simulink model "EX004_FCHEVgasExchange"  (R2023a)
settings: Solver=ode23tb  StartTime=0.0  StopTime=20e3  MaxStep=1e-1  RelTol=1e-4
libraries: component_lib x23, slpidlib x4, simulink x1, base_lib x1
settings Model: Creator=maxjo65  LastModifiedBy=maxjo
settings OptimizationCC: ReuseModelBlockBuffer=off
settings DebuggingCC: UnconnectedInputMsg=warning  UnconnectedOutputMsg=warning  UnconnectedLineMsg=warning
settings ModelReferenceCC: EnableRefExpFcnMdlSchedulingChecks=on
settings RTWCC: DLArmComputeVersion=19.05

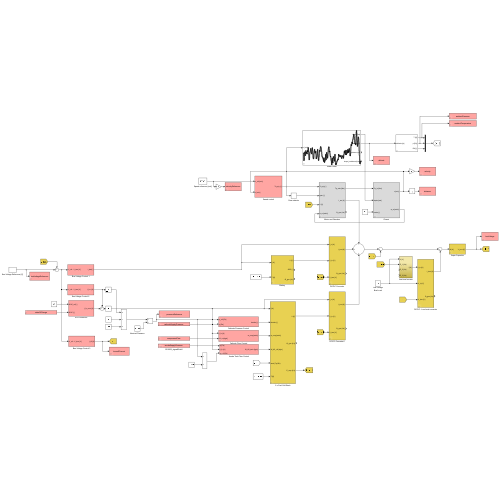
[thumbnail: Simulink's stored preview of the top-level diagram]
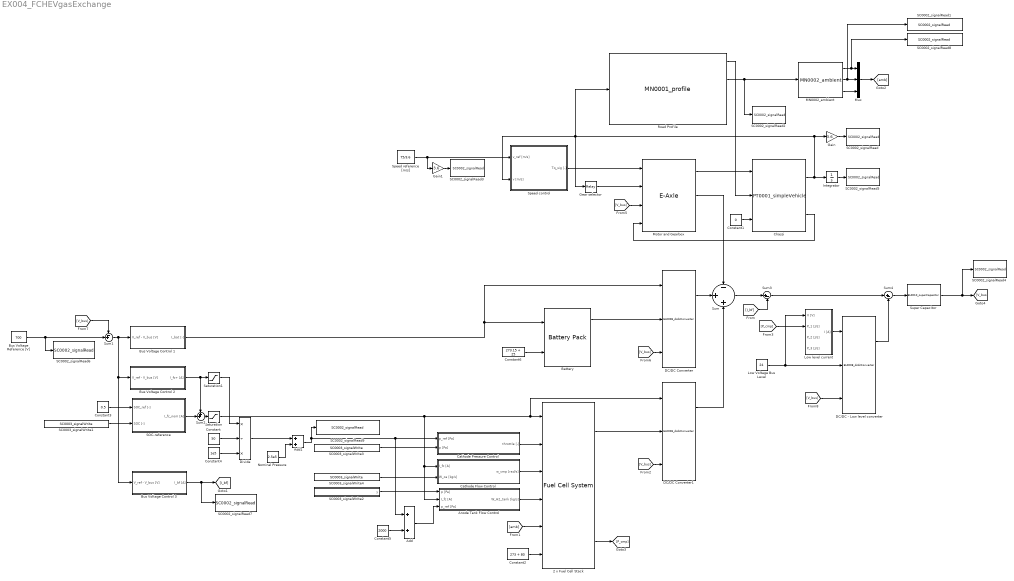
== system EX004_FCHEVgasExchange ==
  2 x Fuel Cell Stack : component_lib/Fuel Cell System  n_st=2  n=375
  Add : Sum
  Add1 : Sum
  Anode Tank Flow Control : Subsystem  mask{n_cell=375}
      mask prompts: n_cell "Cells [-]"
  Battery : component_lib/Battery Pack  SOC_0=0.5  Nx=120  Ny=180
  Bus Voltage Control 1 : Subsystem
  "Bus Voltage Control 2 " : Subsystem
  Bus Voltage Control 3 : Subsystem
  Bus Voltage Reference [V] : Constant  Value=700
  Cathode Flow Control : Subsystem  mask{lambda_O2_ref=2, n_cell=375}
      mask prompts: lambda_O2_ref "Oxygen stoich. reference [-]:"; n_cell "Cells [-]:"
  Cathode Pressure Control : Subsystem
  Chassi : component_lib/Powertrain/PT0001_simpleVehicle  m=40e3  r_w=0.5  A_f=10  C_d=0.5  rho_air=1.225  c_r0=0.0060  c_r1=2.3e-7  gain=600  v0=75/3.6  x0=0
  Constant : Constant  Value=50
  Constant1 : Constant  Value=0
  Constant2 : Constant  Value=273 + 80
  Constant3 : Constant  Value=0.5
  Constant4 : Constant  Value=1e5
  Constant5 : Constant  Value=2000
  Constant6 : Constant  Value=273.15 + 25
  DC/DC - Low level converter : component_lib/Electrochemistry/EL0008_dcdcConverter  eta_up=0.99  eta_down=0.99
  DC/DC Converter : component_lib/Electrochemistry/EL0008_dcdcConverter  eta_up=0.99  eta_down=0.99
  DC/DC Converter1 : component_lib/Electrochemistry/EL0008_dcdcConverter  eta_up=0.99  eta_down=0.99
  Divide : Product  Inputs=*/*
  Gain : Gain  Gain=3.6
  Gain1 : Gain  Gain=3.6
  Gear selector : Relay  OnSwitchValue=22  OffSwitchValue=21.5  OnOutputValue=4  OffOutputValue=3
  Integrator : Integrator
  Low Voltage Bus Level : Constant  Value=24
  Low level current : Subsystem
  MN0002_ambient : component_lib/Mission/MN0002_ambient  p_0=1.01e5  T_0=273 + 20  RH_0=0.05
  Motor and Gearbox : component_lib/E-Axle  n=3  V_nom=700
  Mux : Mux  Inputs=3
  Nominal Pressure : Constant  Value=2.5e5
  Road Profile : component_lib/Mission/MN0001_profile  profile=Sodertalje_Norrkoping.mat  x0=0  N_lookahead=100
  SC0002_signalRead : component_lib/Data & Control/SC0002_signalRead  SigName=velocity
  SC0002_signalRead1 : component_lib/Data & Control/SC0002_signalRead  SigName=ambientPressure
  SC0002_signalRead2 : component_lib/Data & Control/SC0002_signalRead  SigName=altitude
  SC0002_signalRead3 : component_lib/Data & Control/SC0002_signalRead  SigName=velocityReference
  SC0002_signalRead4 : component_lib/Data & Control/SC0002_signalRead  SigName=busVoltage
  SC0002_signalRead5 : component_lib/Data & Control/SC0002_signalRead  SigName=distance
  SC0002_signalRead6 : component_lib/Data & Control/SC0002_signalRead  SigName=busVoltageReference
  SC0002_signalRead7 : component_lib/Data & Control/SC0002_signalRead  SigName=burnoffCurrent
  SC0002_signalRead8 : component_lib/Data & Control/SC0002_signalRead  SigName=ambientTemperature
  SC0002_signalRead9 : component_lib/Data & Control/SC0002_signalRead  SigName=pressureReference
  SC0003_signalWrite1 : component_lib/Data & Control/SC0003_signalWrite  SigName=stateOfCharge
  SC0003_signalWrite2 : Subsystem  AncestorBlock=component_lib/Data & Control/SC0003_signalWrite  mask{SigName=anodeSupplyPressure}
      mask prompts: SigName "Signal identifier:"
      mask init:
      | % set signal name in goto tag
      | set_param([gcb, '/', 'From'], 'GotoTag', SigName)
      settings: LibrarySourceBlock=component_lib/Data & Control/SC0003_signalWrite
      mask Display: disp(SigName)
  SC0003_signalWrite3 : component_lib/Data & Control/SC0003_signalWrite  SigName=cathodeSupplyPressure
  SC0003_signalWrite4 : component_lib/Data & Control/SC0003_signalWrite  SigName=compressorFlow
  SOC-reference : Subsystem
  Saturation : Saturate  UpperLimit=600  LowerLimit=20
  Saturation1 : Saturate  UpperLimit=50  LowerLimit=0
  Speed control : Subsystem
  Speed reference [m/s] : Constant  Value=75/3.6
  Sum : Sum  Inputs=-++
  Sum1 : Sum  Inputs=-+|
  Sum2 : Sum  Inputs=++|
  Sum3 : Sum  Inputs=|+-
  Sum4 : Sum  Inputs=|+-
  Super Capacitor : component_lib/Electrochemistry/EL0010_superCapacitor  C=1  V_bus0=700
  wires:
  Motor and Gearbox/1 -> Chassi/1
  Chassi/2 -> Motor and Gearbox/4
  Road Profile/1 -> Chassi/2
  Chassi/1 -> Integrator/1, Gain/1, Speed control/2(v [m/s]), Road Profile/1, Gear selector/1
  Speed reference [m/s]/1 -> Gain1/1, Speed control/1(v_ref [m/s])
  Speed control/1(Tq_sig [-]) -> Motor and Gearbox/1
  Gear selector/1 -> Motor and Gearbox/2
  Integrator/1 -> SC0002_signalRead5/1
  Gain/1 -> SC0002_signalRead/1
  Road Profile/2 -> MN0002_ambient/1, SC0002_signalRead2/1
  Gain1/1 -> SC0002_signalRead3/1
  Super Capacitor/1 -> SC0002_signalRead4/1, [V_bus]
  Constant1/1 -> Chassi/3
  Battery/1 -> DC/DC Converter/2
  DC/DC Converter/1 -> Sum/2
  Motor and Gearbox/2 -> Sum/1
  Bus Voltage Control 1/1(I_bat [-]) -> DC/DC Converter/1, Battery/1
  DC/DC Converter1/1 -> Sum/3
  Bus Voltage Reference [V]/1 -> Sum1/2, SC0002_signalRead6/1
  Constant3/1 -> SOC-reference/1(SOC_ref [-])
  Sum1/1 -> Bus Voltage Control 3/1(V_ref - V_bus [V]), "Bus Voltage Control 2 "/1(V_ref - V_bus [V]), Bus Voltage Control 1/1(V_ref - V_bus [V])
  Sum2/1 -> Saturation/1
  "Bus Voltage Control 2 "/1(I_fc+ [A]) -> Saturation1/1, Sum2/1
  SOC-reference/1(I_fc_nom [A]) -> Sum2/2
  Sum/1 -> Sum3/1
  Bus Voltage Control 3/1(I_bf [A]) -> SC0002_signalRead7/1, [I_bf]
  [I_bf] -> Sum3/2
  MN0002_ambient/3 -> Mux/3
  Mux/1 -> [amb]
  2 x Fuel Cell Stack/1 -> DC/DC Converter1/2
  2 x Fuel Cell Stack/3 -> [P_cmp]
  Sum3/1 -> Sum4/1
  Sum4/1 -> Super Capacitor/1
  DC/DC - Low level converter/1 -> Sum4/2
  [P_cmp] -> Low level current/2(P_1 [J/s])
  Low Voltage Bus Level/1 -> Low level current/1(V [V]), DC/DC - Low level converter/2
  [V_bus] -> Motor and Gearbox/3
  [V_bus] -> Sum1/1
  Cathode Flow Control/1(w_cmp [rad/s]) -> 2 x Fuel Cell Stack/3
  SC0003_signalWrite4/1 -> Cathode Flow Control/2(W_ca [kg/s])
  Cathode Pressure Control/1(throttle [-]) -> 2 x Fuel Cell Stack/2
  SC0003_signalWrite3/1 -> Cathode Pressure Control/2(p [Pa])
  SC0003_signalWrite2/1(y) -> Anode Tank Flow Control/1(p [Pa])
  Add1/1 -> Add/1, Cathode Pressure Control/1(p_ref [Pa]), SC0002_signalRead9/1
  Anode Tank Flow Control/1(W_H2_tank [kg/s]) -> 2 x Fuel Cell Stack/4
  Add/1 -> Anode Tank Flow Control/3(p_ref [Pa])
  Constant5/1 -> Add/2
  Saturation/1 -> Anode Tank Flow Control/2(I_fc [A]), Cathode Flow Control/1(I_fc [A]), DC/DC Converter1/1, 2 x Fuel Cell Stack/1
  Constant2/1 -> 2 x Fuel Cell Stack/6
  [amb] -> 2 x Fuel Cell Stack/5
  SC0003_signalWrite1/1 -> SOC-reference/2(SOC [-])
  MN0002_ambient/2 -> Mux/2, SC0002_signalRead1/1
  MN0002_ambient/1 -> SC0002_signalRead8/1, Mux/1
  Constant/1 -> Divide/2
  Constant4/1 -> Divide/3
  Nominal Pressure/1 -> Add1/2
  Saturation1/1 -> Divide/1
  Divide/1 -> Add1/1
  [V_bus] -> DC/DC Converter/3
  Constant6/1 -> Battery/2
  [V_bus] -> DC/DC Converter1/3
  Low level current/1(I [A]) -> DC/DC - Low level converter/1
  [V_bus] -> DC/DC - Low level converter/3

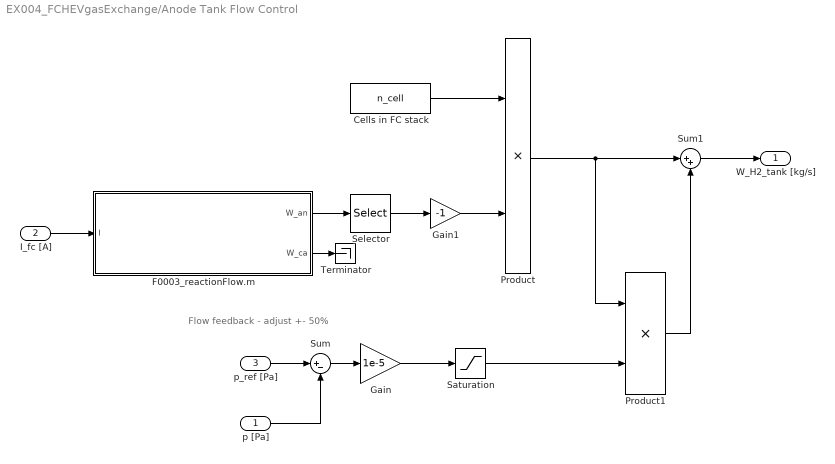
== system EX004_FCHEVgasExchange/Anode Tank Flow Control ==
  note: Flow feedback - adjust +- 50%
  p [Pa] : Inport
  I_fc [A] : Inport  Port=2
  p_ref [Pa] : Inport  Port=3
  Cells in FC stack : Constant  Value=n_cell
  F0003_reactionFlow.m : MATLAB Function  TreatAsAtomicUnit=on
  Gain : Gain  Gain=1e-5
  Gain1 : Gain  Gain=-1
  Product : Product
  Product1 : Product
  Saturation : Saturate
  Selector : Selector  InputPortWidth=4  IndexOptions=Index vector (dialog)  Indices=1  OutputSizes=1
  Sum : Sum  Inputs=|+-
  Sum1 : Sum  Inputs=|++
  Terminator : Terminator
  W_H2_tank [kg/s] : Outport
  wires:
  Product1/1 -> Sum1/2
  Sum/1 -> Gain/1
  Sum1/1 -> W_H2_tank [kg/s]/1
  Product/1 -> Product1/1, Sum1/1
  p [Pa]/1 -> Sum/2
  p_ref [Pa]/1 -> Sum/1
  Cells in FC stack/1 -> Product/1
  F0003_reactionFlow.m/2(W_ca) -> Terminator/1
  I_fc [A]/1 -> F0003_reactionFlow.m/1(I)
  F0003_reactionFlow.m/1(W_an) -> Selector/1
  Selector/1 -> Gain1/1
  Gain1/1 -> Product/2
  Gain/1 -> Saturation/1
  Saturation/1 -> Product1/2

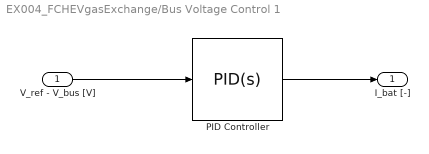
== system EX004_FCHEVgasExchange/Bus Voltage Control 1 ==
  V_ref - V_bus [V] : Inport
  PID Controller : slpidlib/PID Controller  Controller=PID  Form=Parallel  TimeDomain=Continuous-time  UseExternalTs=off  SampleTime=-1  IntegratorMethod=Forward Euler  FilterMethod=Forward Euler  ControllerParametersSource=internal  P=1e2  I=1  UseKiTs=off  D=0  N=100  UseFilter=on  TunerSelectOption=Transfer Function Based (PID Tuner App)  ZeroCross=off  InitialConditionSource=internal  InitialConditionForIntegrator=0  InitialConditionForFilter=0  DifferentiatorICPrevScaledInput=0  ExternalReset=none  TrackingMode=off  Kt=1  LimitOutput=on  SatLimitsSource=internal  UpperSaturationLimit=350  LowerSaturationLimit=-350  LinearizeAsGain=on  AntiWindupMode=clamping  Kb=1  LimitIntegrator=off  UpperIntegratorSaturationLimit=inf  LowerIntegratorSaturationLimit=-inf  POutMin=[]  POutMax=[]  IOutMin=[]  IOutMax=[]  DOutMin=[]  DOutMax=[]  NOutMin=[]  NOutMax=[]  SumOutMin=[]  SumOutMax=[]  SaturationOutMin=[]  SaturationOutMax=[]  PParamMin=[]  PParamMax=[]  IParamMin=[]  IParamMax=[]  DParamMin=[]  DParamMax=[]  NParamMin=[]  NParamMax=[]  KbParamMin=[]  KbParamMax=[]  KtParamMin=[]  KtParamMax=[]  KbOutMin=[]  KbOutMax=[]  KtOutMin=[]  KtOutMax=[]  IntegratorOutMin=[]  IntegratorOutMax=[]  FilterOutMin=[]  FilterOutMax=[]  SumI1OutMin=[]  SumI1OutMax=[]  SumI2OutMin=[]  SumI2OutMax=[]  SumI3OutMin=[]  SumI3OutMax=[]  SumI4OutMin=[]  SumI4OutMax=[]  SumDOutMin=[]  SumDOutMax=[]  DifferentiatorOutMin=[]  DifferentiatorOutMax=[]  FilterDiffOutCoefMin=[]  FilterDiffOutCoefMax=[]  ReciprocalOutMin=[]  ReciprocalOutMax=[]  SumDenOutMin=[]  SumDenOutMax=[]  SumNumOutMin=[]  SumNumOutMax=[]  DivideOutMin=[]  DivideOutMax=[]  UdiffTsProdOutMin=[]  UdiffTsProdOutMax=[]  NTsProdOutMin=[]  NTsProdOutMax=[]  UintegralTsProdOutMin=[]  UintegralTsProdOutMax=[]  UngainTsProdOutMin=[]  UngainTsProdOutMax=[]  ClampingZeroOutDataTypeStr=Inherit: Inherit via back propagation  ClampingZeroOutMin=[]  ClampingZeroOutMax=[]  FilterDenConstantOutDataTypeStr=Inherit: Inherit via back propagation  FilterDenConstantOutMin=[]  FilterDenConstantOutMax=[]  PCopyOutDataTypeStr=Inherit: Inherit via back propagation  PCopyOutMin=[]  PCopyOutMax=[]  NCopyOutDataTypeStr=Inherit: Inherit via back propagation  NCopyOutMin=[]  NCopyOutMax=[]  IntegratorContinuousStateAttributes=''  IntegratorStateMustResolveToSignalObject=off  IntegratorRTWStateStorageClass=Auto  FilterContinuousStateAttributes=''  FilterStateMustResolveToSignalObject=off  FilterRTWStateStorageClass=Auto  ParallelPVariant=InternalParameters  IdealPVariant=Disabled  IVariant=InternalParameters  DVariant=InternalParameters  IntegratorVariant=Continuous  SatVariant=Enabled  AWVariant=ContClampingParallel  PCopyVariant=Disabled  TRVariant=Disabled  FdbkBlocksVariant=Forward  IdealPFdbkVariant=Disabled  SatFdbkVariant=Disabled  DerivativeFilterVariant=ContFilter  NVariant=InternalParameters  NCopyVariant=Disabled  FilterICVariant=InternalICsFilter  IntegratorICVariant=InternalICs  ExternalResetVariant=Disabled  TRSumVariant=Passthrough  SumFdbkVariant=Disabled  SumVariant=Sum_PID  TsampFilterVariant=InternalTs  TsampNgainVariant=Passthrough  TsampIntegralVariant=Disabled_SignalSpec  ExternalSaturationOutDataTypeStr=Inherit: Same as second input
  I_bat [-] : Outport
  wires:
  PID Controller/1 -> I_bat [-]/1
  V_ref - V_bus [V]/1 -> PID Controller/1

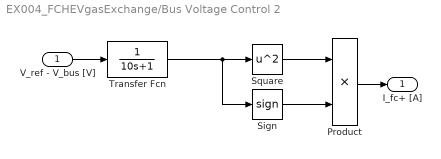
== system EX004_FCHEVgasExchange/Bus Voltage Control 2  ==
  V_ref - V_bus [V] : Inport
  Product : Product
  Sign : Signum
  Square : Math  Operator=square
  Transfer Fcn : TransferFcn  Denominator=[10 1]
  I_fc+ [A] : Outport
  wires:
  Sign/1 -> Product/2
  Transfer Fcn/1 -> Sign/1, Square/1
  Square/1 -> Product/1
  V_ref - V_bus [V]/1 -> Transfer Fcn/1
  Product/1 -> I_fc+ [A]/1

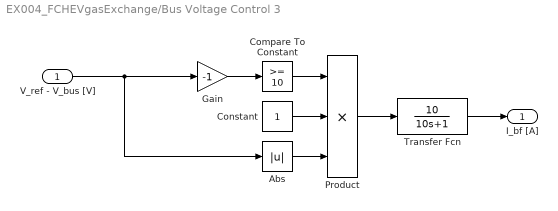
== system EX004_FCHEVgasExchange/Bus Voltage Control 3 ==
  V_ref - V_bus [V] : Inport
  Abs : Abs  SaturateOnIntegerOverflow=off
  Compare To Constant : simulink/Logic and Bit Operations/Compare To Constant  relop=>=  const=10  OutDataTypeStr=boolean
  Constant : Constant
  Gain : Gain  Gain=-1
  Product : Product  Inputs=3
  Transfer Fcn : TransferFcn  Numerator=[10]  Denominator=[10 1]
  I_bf [A] : Outport
  wires:
  Gain/1 -> Compare To Constant/1
  Transfer Fcn/1 -> I_bf [A]/1
  Compare To Constant/1 -> Product/1
  Product/1 -> Transfer Fcn/1
  V_ref - V_bus [V]/1 -> Abs/1, Gain/1
  Abs/1 -> Product/3
  Constant/1 -> Product/2

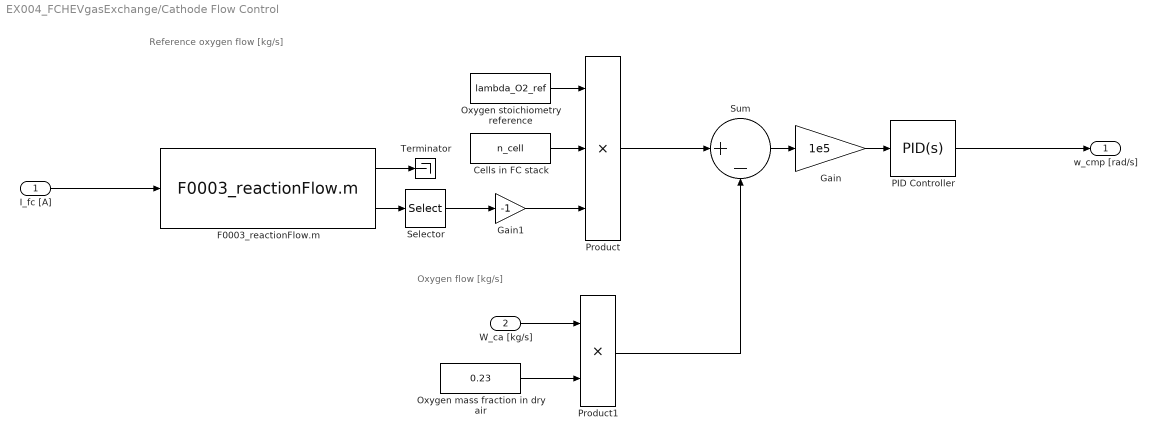
== system EX004_FCHEVgasExchange/Cathode Flow Control ==
  note: Reference oxygen flow [kg/s]
  note: Oxygen flow [kg/s]
  I_fc [A] : Inport
  W_ca [kg/s] : Inport  Port=2
  Cells in FC stack : Constant  Value=n_cell
  F0003_reactionFlow.m : base_lib/F0003_pukrushpan2004/F0003_reactionFlow.m  SystemSampleTime=-1  VariantActivationTime=update diagram  Latency=0  AutoFrameSizeCalculation=off
      settings: LibrarySourceBlock=|
      | simulink/User-Defined
      | Functions/MATLAB Function
  Gain : Gain  Gain=1e5
  Gain1 : Gain  Gain=-1
  Oxygen mass fraction in dry air : Constant  Value=0.23
  Oxygen stoichiometry reference : Constant  Value=lambda_O2_ref
  PID Controller : slpidlib/PID Controller  Controller=PID  Form=Parallel  TimeDomain=Continuous-time  UseExternalTs=off  SampleTime=-1  IntegratorMethod=Forward Euler  FilterMethod=Forward Euler  ControllerParametersSource=internal  P=30  I=0.7  UseKiTs=off  D=0  N=100  UseFilter=on  TunerSelectOption=Transfer Function Based (PID Tuner App)  ZeroCross=off  InitialConditionSource=internal  InitialConditionForIntegrator=10e3  InitialConditionForFilter=10e3  DifferentiatorICPrevScaledInput=0  ExternalReset=none  TrackingMode=off  Kt=1  LimitOutput=on  SatLimitsSource=internal  UpperSaturationLimit=20e3  LowerSaturationLimit=3e3  LinearizeAsGain=on  AntiWindupMode=clamping  Kb=1e-1  LimitIntegrator=off  UpperIntegratorSaturationLimit=inf  LowerIntegratorSaturationLimit=-inf  POutMin=[]  POutMax=[]  IOutMin=[]  IOutMax=[]  DOutMin=[]  DOutMax=[]  NOutMin=[]  NOutMax=[]  SumOutMin=[]  SumOutMax=[]  SaturationOutMin=[]  SaturationOutMax=[]  PParamMin=[]  PParamMax=[]  IParamMin=[]  IParamMax=[]  DParamMin=[]  DParamMax=[]  NParamMin=[]  NParamMax=[]  KbParamMin=[]  KbParamMax=[]  KtParamMin=[]  KtParamMax=[]  KbOutMin=[]  KbOutMax=[]  KtOutMin=[]  KtOutMax=[]  IntegratorOutMin=[]  IntegratorOutMax=[]  FilterOutMin=[]  FilterOutMax=[]  SumI1OutMin=[]  SumI1OutMax=[]  SumI2OutMin=[]  SumI2OutMax=[]  SumI3OutMin=[]  SumI3OutMax=[]  SumI4OutMin=[]  SumI4OutMax=[]  SumDOutMin=[]  SumDOutMax=[]  DifferentiatorOutMin=[]  DifferentiatorOutMax=[]  FilterDiffOutCoefMin=[]  FilterDiffOutCoefMax=[]  ReciprocalOutMin=[]  ReciprocalOutMax=[]  SumDenOutMin=[]  SumDenOutMax=[]  SumNumOutMin=[]  SumNumOutMax=[]  DivideOutMin=[]  DivideOutMax=[]  UdiffTsProdOutMin=[]  UdiffTsProdOutMax=[]  NTsProdOutMin=[]  NTsProdOutMax=[]  UintegralTsProdOutMin=[]  UintegralTsProdOutMax=[]  UngainTsProdOutMin=[]  UngainTsProdOutMax=[]  ClampingZeroOutDataTypeStr=Inherit: Inherit via back propagation  ClampingZeroOutMin=[]  ClampingZeroOutMax=[]  FilterDenConstantOutDataTypeStr=Inherit: Inherit via back propagation  FilterDenConstantOutMin=[]  FilterDenConstantOutMax=[]  PCopyOutDataTypeStr=Inherit: Inherit via back propagation  PCopyOutMin=[]  PCopyOutMax=[]  NCopyOutDataTypeStr=Inherit: Inherit via back propagation  NCopyOutMin=[]  NCopyOutMax=[]  IntegratorContinuousStateAttributes=''  IntegratorStateMustResolveToSignalObject=off  IntegratorRTWStateStorageClass=Auto  FilterContinuousStateAttributes=''  FilterStateMustResolveToSignalObject=off  FilterRTWStateStorageClass=Auto  ParallelPVariant=InternalParameters  IdealPVariant=Disabled  IVariant=InternalParameters  DVariant=InternalParameters  IntegratorVariant=Continuous  SatVariant=Enabled  AWVariant=ContClampingParallel  PCopyVariant=Disabled  TRVariant=Disabled  FdbkBlocksVariant=Forward  IdealPFdbkVariant=Disabled  SatFdbkVariant=Disabled  DerivativeFilterVariant=ContFilter  NVariant=InternalParameters  NCopyVariant=Disabled  FilterICVariant=InternalICsFilter  IntegratorICVariant=InternalICs  ExternalResetVariant=Disabled  TRSumVariant=Passthrough  SumFdbkVariant=Disabled  SumVariant=Sum_PID  TsampFilterVariant=InternalTs  TsampNgainVariant=Passthrough  TsampIntegralVariant=Disabled_SignalSpec  ExternalSaturationOutDataTypeStr=Inherit: Same as second input
  Product : Product  Inputs=3
  Product1 : Product
  Selector : Selector  InputPortWidth=4  IndexOptions=Index vector (dialog)  Indices=2  OutputSizes=1
  Sum : Sum  Inputs=|+-
  Terminator : Terminator
  w_cmp [rad/s] : Outport
  wires:
  W_ca [kg/s]/1 -> Product1/1
  I_fc [A]/1 -> F0003_reactionFlow.m/1
  Gain/1 -> PID Controller/1
  PID Controller/1 -> w_cmp [rad/s]/1
  Sum/1 -> Gain/1
  Product1/1 -> Sum/2
  Product/1 -> Sum/1
  Cells in FC stack/1 -> Product/2
  Gain1/1 -> Product/3
  F0003_reactionFlow.m/1 -> Terminator/1
  Oxygen mass fraction in dry air/1 -> Product1/2
  Selector/1 -> Gain1/1
  Oxygen stoichiometry reference/1 -> Product/1
  F0003_reactionFlow.m/2 -> Selector/1

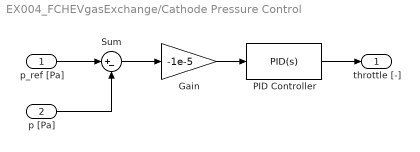
== system EX004_FCHEVgasExchange/Cathode Pressure Control ==
  p_ref [Pa] : Inport
  p [Pa] : Inport  Port=2
  Gain : Gain  Gain=-1e-5
  PID Controller : slpidlib/PID Controller  Controller=PID  Form=Parallel  TimeDomain=Continuous-time  UseExternalTs=off  SampleTime=-1  IntegratorMethod=Forward Euler  FilterMethod=Forward Euler  ControllerParametersSource=internal  P=1  I=1e-1  UseKiTs=off  D=0  N=100  UseFilter=on  TunerSelectOption=Transfer Function Based (PID Tuner App)  ZeroCross=off  InitialConditionSource=internal  InitialConditionForIntegrator=0.5  InitialConditionForFilter=0.5  DifferentiatorICPrevScaledInput=0  ExternalReset=none  TrackingMode=off  Kt=1  LimitOutput=on  SatLimitsSource=internal  UpperSaturationLimit=0.99  LowerSaturationLimit=0.01  LinearizeAsGain=on  AntiWindupMode=clamping  Kb=1  LimitIntegrator=off  UpperIntegratorSaturationLimit=inf  LowerIntegratorSaturationLimit=-inf  POutMin=[]  POutMax=[]  IOutMin=[]  IOutMax=[]  DOutMin=[]  DOutMax=[]  NOutMin=[]  NOutMax=[]  SumOutMin=[]  SumOutMax=[]  SaturationOutMin=[]  SaturationOutMax=[]  PParamMin=[]  PParamMax=[]  IParamMin=[]  IParamMax=[]  DParamMin=[]  DParamMax=[]  NParamMin=[]  NParamMax=[]  KbParamMin=[]  KbParamMax=[]  KtParamMin=[]  KtParamMax=[]  KbOutMin=[]  KbOutMax=[]  KtOutMin=[]  KtOutMax=[]  IntegratorOutMin=[]  IntegratorOutMax=[]  FilterOutMin=[]  FilterOutMax=[]  SumI1OutMin=[]  SumI1OutMax=[]  SumI2OutMin=[]  SumI2OutMax=[]  SumI3OutMin=[]  SumI3OutMax=[]  SumI4OutMin=[]  SumI4OutMax=[]  SumDOutMin=[]  SumDOutMax=[]  DifferentiatorOutMin=[]  DifferentiatorOutMax=[]  FilterDiffOutCoefMin=[]  FilterDiffOutCoefMax=[]  ReciprocalOutMin=[]  ReciprocalOutMax=[]  SumDenOutMin=[]  SumDenOutMax=[]  SumNumOutMin=[]  SumNumOutMax=[]  DivideOutMin=[]  DivideOutMax=[]  UdiffTsProdOutMin=[]  UdiffTsProdOutMax=[]  NTsProdOutMin=[]  NTsProdOutMax=[]  UintegralTsProdOutMin=[]  UintegralTsProdOutMax=[]  UngainTsProdOutMin=[]  UngainTsProdOutMax=[]  ClampingZeroOutDataTypeStr=Inherit: Inherit via back propagation  ClampingZeroOutMin=[]  ClampingZeroOutMax=[]  FilterDenConstantOutDataTypeStr=Inherit: Inherit via back propagation  FilterDenConstantOutMin=[]  FilterDenConstantOutMax=[]  PCopyOutDataTypeStr=Inherit: Inherit via back propagation  PCopyOutMin=[]  PCopyOutMax=[]  NCopyOutDataTypeStr=Inherit: Inherit via back propagation  NCopyOutMin=[]  NCopyOutMax=[]  IntegratorContinuousStateAttributes=''  IntegratorStateMustResolveToSignalObject=off  IntegratorRTWStateStorageClass=Auto  FilterContinuousStateAttributes=''  FilterStateMustResolveToSignalObject=off  FilterRTWStateStorageClass=Auto  ParallelPVariant=InternalParameters  IdealPVariant=Disabled  IVariant=InternalParameters  DVariant=InternalParameters  IntegratorVariant=Continuous  SatVariant=Enabled  AWVariant=ContClampingParallel  PCopyVariant=Disabled  TRVariant=Disabled  FdbkBlocksVariant=Forward  IdealPFdbkVariant=Disabled  SatFdbkVariant=Disabled  DerivativeFilterVariant=ContFilter  NVariant=InternalParameters  NCopyVariant=Disabled  FilterICVariant=InternalICsFilter  IntegratorICVariant=InternalICs  ExternalResetVariant=Disabled  TRSumVariant=Passthrough  SumFdbkVariant=Disabled  SumVariant=Sum_PID  TsampFilterVariant=InternalTs  TsampNgainVariant=Passthrough  TsampIntegralVariant=Disabled_SignalSpec  ExternalSaturationOutDataTypeStr=Inherit: Same as second input
  Sum : Sum  Inputs=|+-
  throttle [-] : Outport
  wires:
  Sum/1 -> Gain/1
  p [Pa]/1 -> Sum/2
  Gain/1 -> PID Controller/1
  PID Controller/1 -> throttle [-]/1
  p_ref [Pa]/1 -> Sum/1

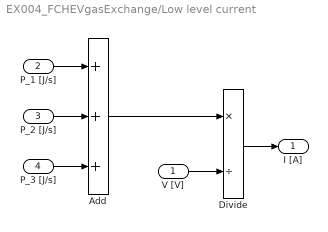
== system EX004_FCHEVgasExchange/Low level current ==
  V [V] : Inport
  P_1 [J/s] : Inport  Port=2
  P_2 [J/s] : Inport  Port=3
  P_3 [J/s] : Inport  Port=4
  Add : Sum  Inputs=+++
  Divide : Product  Inputs=*/
  I [A] : Outport
  wires:
  Add/1 -> Divide/1
  P_1 [J/s]/1 -> Add/1
  V [V]/1 -> Divide/2
  P_3 [J/s]/1 -> Add/3
  P_2 [J/s]/1 -> Add/2
  Divide/1 -> I [A]/1

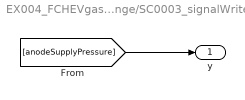
== system EX004_FCHEVgasExchange/SC0003_signalWrite2 ==
  y : Outport
  wires:
  [anodeSupplyPressure] -> y/1

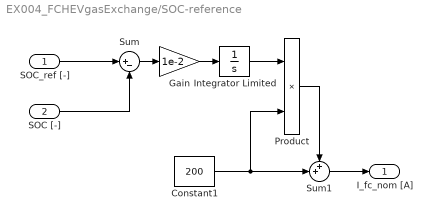
== system EX004_FCHEVgasExchange/SOC-reference ==
  SOC_ref [-] : Inport
  SOC [-] : Inport  Port=2
  Constant1 : Constant  Value=200
  Gain : Gain  Gain=1e-2
  Integrator Limited : Integrator  LimitOutput=on  UpperSaturationLimit=1  LowerSaturationLimit=-1
  Product : Product
  Sum : Sum  Inputs=|+-
  Sum1 : Sum  Inputs=++|
  I_fc_nom [A] : Outport
  wires:
  Product/1 -> Sum1/1
  Integrator Limited/1 -> Product/1
  Sum1/1 -> I_fc_nom [A]/1
  Constant1/1 -> Sum1/2, Product/2
  Sum/1 -> Gain/1
  SOC [-]/1 -> Sum/2
  Gain/1 -> Integrator Limited/1
  SOC_ref [-]/1 -> Sum/1

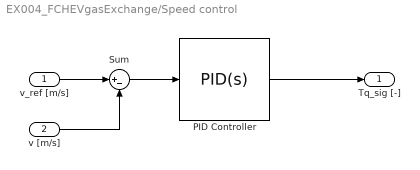
== system EX004_FCHEVgasExchange/Speed control ==
  v_ref [m/s] : Inport
  v [m/s] : Inport  Port=2
  PID Controller : slpidlib/PID Controller  Controller=PID  Form=Parallel  TimeDomain=Continuous-time  UseExternalTs=off  SampleTime=-1  IntegratorMethod=Forward Euler  FilterMethod=Forward Euler  ControllerParametersSource=internal  P=10  I=1e-1  UseKiTs=off  D=0  N=100  UseFilter=on  TunerSelectOption=Transfer Function Based (PID Tuner App)  ZeroCross=off  InitialConditionSource=internal  InitialConditionForIntegrator=0  InitialConditionForFilter=0  DifferentiatorICPrevScaledInput=0  ExternalReset=none  TrackingMode=off  Kt=1  LimitOutput=on  SatLimitsSource=internal  UpperSaturationLimit=1  LowerSaturationLimit=-1  LinearizeAsGain=on  AntiWindupMode=clamping  Kb=1  LimitIntegrator=off  UpperIntegratorSaturationLimit=inf  LowerIntegratorSaturationLimit=-inf  POutMin=[]  POutMax=[]  IOutMin=[]  IOutMax=[]  DOutMin=[]  DOutMax=[]  NOutMin=[]  NOutMax=[]  SumOutMin=[]  SumOutMax=[]  SaturationOutMin=[]  SaturationOutMax=[]  PParamMin=[]  PParamMax=[]  IParamMin=[]  IParamMax=[]  DParamMin=[]  DParamMax=[]  NParamMin=[]  NParamMax=[]  KbParamMin=[]  KbParamMax=[]  KtParamMin=[]  KtParamMax=[]  KbOutMin=[]  KbOutMax=[]  KtOutMin=[]  KtOutMax=[]  IntegratorOutMin=[]  IntegratorOutMax=[]  FilterOutMin=[]  FilterOutMax=[]  SumI1OutMin=[]  SumI1OutMax=[]  SumI2OutMin=[]  SumI2OutMax=[]  SumI3OutMin=[]  SumI3OutMax=[]  SumI4OutMin=[]  SumI4OutMax=[]  SumDOutMin=[]  SumDOutMax=[]  DifferentiatorOutMin=[]  DifferentiatorOutMax=[]  FilterDiffOutCoefMin=[]  FilterDiffOutCoefMax=[]  ReciprocalOutMin=[]  ReciprocalOutMax=[]  SumDenOutMin=[]  SumDenOutMax=[]  SumNumOutMin=[]  SumNumOutMax=[]  DivideOutMin=[]  DivideOutMax=[]  UdiffTsProdOutMin=[]  UdiffTsProdOutMax=[]  NTsProdOutMin=[]  NTsProdOutMax=[]  UintegralTsProdOutMin=[]  UintegralTsProdOutMax=[]  UngainTsProdOutMin=[]  UngainTsProdOutMax=[]  ClampingZeroOutDataTypeStr=Inherit: Inherit via back propagation  ClampingZeroOutMin=[]  ClampingZeroOutMax=[]  FilterDenConstantOutDataTypeStr=Inherit: Inherit via back propagation  FilterDenConstantOutMin=[]  FilterDenConstantOutMax=[]  PCopyOutDataTypeStr=Inherit: Inherit via back propagation  PCopyOutMin=[]  PCopyOutMax=[]  NCopyOutDataTypeStr=Inherit: Inherit via back propagation  NCopyOutMin=[]  NCopyOutMax=[]  IntegratorContinuousStateAttributes=''  IntegratorStateMustResolveToSignalObject=off  IntegratorRTWStateStorageClass=Auto  FilterContinuousStateAttributes=''  FilterStateMustResolveToSignalObject=off  FilterRTWStateStorageClass=Auto  ParallelPVariant=InternalParameters  IdealPVariant=Disabled  IVariant=InternalParameters  DVariant=InternalParameters  IntegratorVariant=Continuous  SatVariant=Enabled  AWVariant=ContClampingParallel  PCopyVariant=Disabled  TRVariant=Disabled  FdbkBlocksVariant=Forward  IdealPFdbkVariant=Disabled  SatFdbkVariant=Disabled  DerivativeFilterVariant=ContFilter  NVariant=InternalParameters  NCopyVariant=Disabled  FilterICVariant=InternalICsFilter  IntegratorICVariant=InternalICs  ExternalResetVariant=Disabled  TRSumVariant=Passthrough  SumFdbkVariant=Disabled  SumVariant=Sum_PID  TsampFilterVariant=InternalTs  TsampNgainVariant=Passthrough  TsampIntegralVariant=Disabled_SignalSpec  ExternalSaturationOutDataTypeStr=Inherit: Same as second input
  Sum : Sum  Inputs=|+-
  Tq_sig [-] : Outport
  wires:
  PID Controller/1 -> Tq_sig [-]/1
  Sum/1 -> PID Controller/1
  v_ref [m/s]/1 -> Sum/1
  v [m/s]/1 -> Sum/2

== matlab function EX004_FCHEVgasExchange/Anode Tank Flow Control/F0003_reactionFlow.m ==
  data: I input; W_an output; W_ca output
function [W_an, W_ca] = F0003_reactionFlow(I)
% constants
F     = 96485; % [C/mol]  - Faradays constant
M_H2  = 0.002; % [kg/mol] - hydrogen molecular weight
M_O2  = 0.032; % [kg/mol] - oxygen   molecular weight
% M_N2  = 0.028; % [kg/mol] - nitrogen molecular weight
M_H2O = 0.018; % [kg/mol] - water    molecular weight

% reaction flows
W_H2_rct  = I * M_H2  /(2*F);
W_O2_rct  = I * M_O2  /(4*F);
W_H2O_rct = I * M_H2O /(2*F);

% output
W_an = [-W_H2_rct;         0;         0; 0];
W_ca = [        0; -W_O2_rct; W_H2O_rct; 0]; 
end
